simulink model "DecMPC"  (R2023a)
settings: Solver=VariableStepAuto  StartTime=0.0  StopTime=1000000  RelTol=1e-3
settings Model: Creator=alex  LastModifiedBy=alex

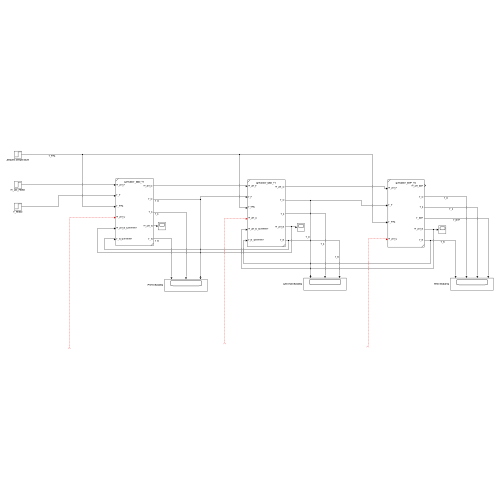
[thumbnail: Simulink's stored preview of the top-level diagram]
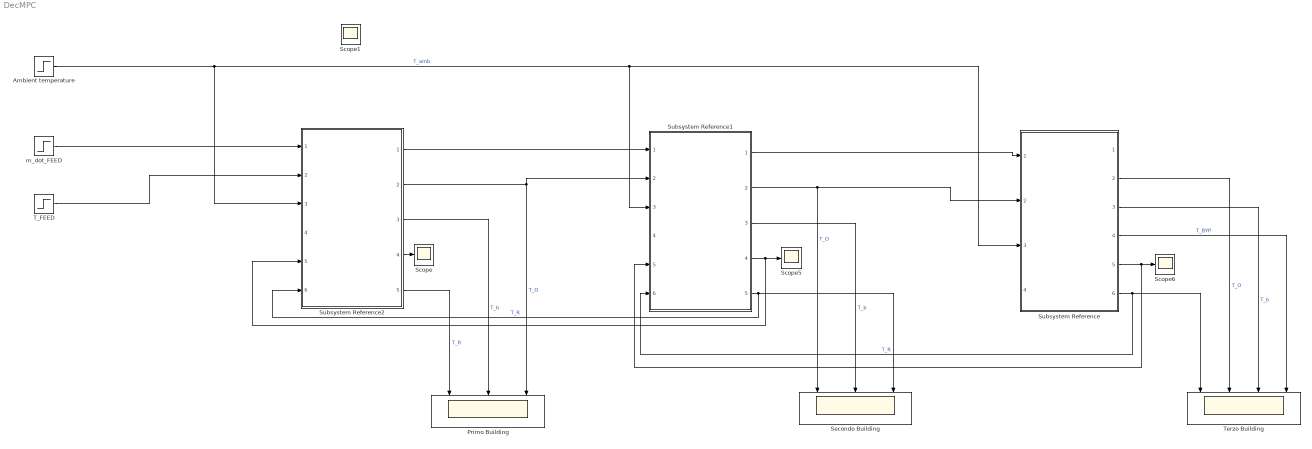
== system DecMPC ==
  Ambient temperature : Step  After=300  SampleTime=0
  Primo Building : Scope  NumInputPorts=3
  Scope{,1,5..6} (4 alike) : Scope
  Secondo Building : Scope  NumInputPorts=3
  Subsystem Reference : Subsystem  ReferencedSubsystem=Simulator_BYP_v0  rho=971  rho_air=971  c_p=4179  c_p_air=4179  pi=3.14151  L_F=40.5  D_F=0.4  h_F=1.5  D_S1=0.1  L_S1=5  h_S1=1.5  D_S2=0.025  L_S2=5000  h_S2=300  D_S3=0.1  L_S3=5  h_S3=1.5  D_R=0.4  L_R=40  h_R=1.5  C_b=100  A_b=500  h_b=1.5  D_BYP=0.1  L_BYP=3  h_BYP=1.5  T_F_0=273  T_S1_0=273  T_S2_0=273  T_S3_0=273  T_b_0=273  T_R_0=273
  Subsystem Reference1 : Subsystem  ReferencedSubsystem=Simulator_MID_v1  rho=971  rho_air=971  c_p=4179  c_p_air=4179  pi=3.14151  L_F=40.5  D_F=0.4  h_F=1.5  D_S1=0.1  L_S1=5  h_S1=1.5  D_S2=0.02  L_S2=50  h_S2=1.5  D_S3=0.1  L_S3=5  h_S3=1.5  D_R=0.4  L_R=40  h_R=1.5  C_b=300  A_b=500  h_b=1.5  T_F_0=273  T_S1_0=273  T_S2_0=273  T_S3_0=273  T_b_0=273  T_R_0=273
  Subsystem Reference2 : Subsystem  ReferencedSubsystem=Simulator_MID_v1  rho=971  rho_air=971  c_p=4179  c_p_air=4179  pi=3.14151  L_F=40.5  D_F=0.4  h_F=1.5  D_S1=0.1  L_S1=5  h_S1=1.5  D_S2=0.02  L_S2=50  h_S2=1.5  D_S3=0.1  L_S3=5  h_S3=1.5  D_R=0.4  L_R=40  h_R=1.5  C_b=300  A_b=500  h_b=1.5  T_F_0=273  T_S1_0=273  T_S2_0=273  T_S3_0=273  T_b_0=273  T_R_0=273
  T_FEED : Step  Time=0  After=350  SampleTime=0
  Terzo Building : Scope  NumInputPorts=4
  m_dot_FEED : Step  Time=0  After=0.1  SampleTime=0
  wires:
  Subsystem Reference1/1 -> Subsystem Reference/1
  Subsystem Reference1/2 -> Secondo Building/1, Subsystem Reference/2  "T_O"
  Ambient temperature/1 -> Subsystem Reference2/3, Subsystem Reference/3, Subsystem Reference1/3  "T_amb"
  Subsystem Reference/6 -> Terzo Building/1, Subsystem Reference1/6  "T_R"
  Subsystem Reference/5 -> Scope6/1, Subsystem Reference1/5
  Subsystem Reference/2 -> Terzo Building/2  "T_O"
  Subsystem Reference/3 -> Terzo Building/3  "T_b"
  Subsystem Reference/4 -> Terzo Building/4  "T_BYP"
  Subsystem Reference1/3 -> Secondo Building/2  "T_b"
  Subsystem Reference1/5 -> Subsystem Reference2/6, Secondo Building/3  "T_R"
  Subsystem Reference2/1 -> Subsystem Reference1/1
  Subsystem Reference2/2 -> Subsystem Reference1/2, Primo Building/3  "T_O"
  Subsystem Reference1/4 -> Scope5/1, Subsystem Reference2/5
  Subsystem Reference2/5 -> Primo Building/1  "T_R"
  Subsystem Reference2/3 -> Primo Building/2  "T_b"
  Subsystem Reference2/4 -> Scope/1
  m_dot_FEED/1 -> Subsystem Reference2/1
  T_FEED/1 -> Subsystem Reference2/2
  ? -> Subsystem Reference2/4
  ? -> Subsystem Reference1/4
  ? -> Subsystem Reference/4
